simulink subsystem "Plant"  (R2024b)
settings: Solver=VariableStepAuto  StartTime=0.0  StopTime=10.0  RelTol=1e-3
undefined symbols (not defined in the file): body, wheels
settings Model: Creator=Marij  LastModifiedBy=marijn

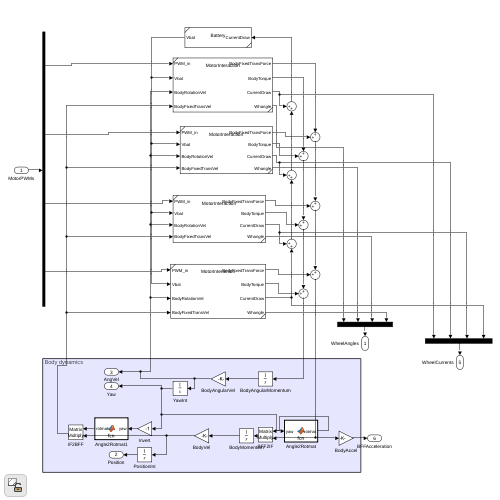
[thumbnail: Simulink's stored preview of the top-level diagram]
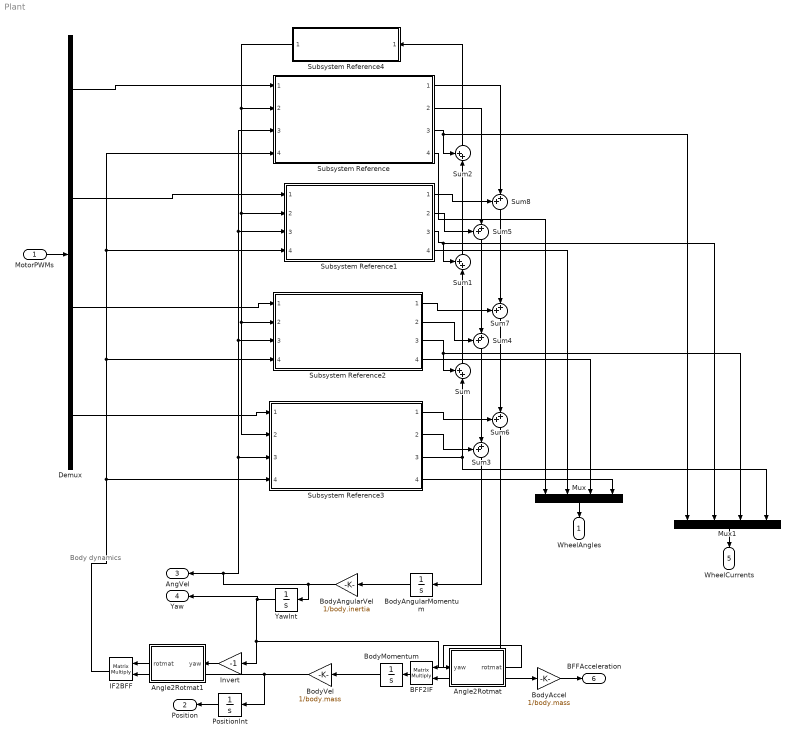
== system Plant ==
  note: Body dynamics
  MotorPWMs : Inport  PortDimensions=4
  Angle2Rotmat : MATLAB Function  TreatAsAtomicUnit=on
  Angle2Rotmat1 : MATLAB Function  TreatAsAtomicUnit=on
  BFF2IF : Product  Multiplication=Matrix(*)
  BodyAccel : Gain  Gain=1/body.mass
  BodyAngularMomentum : Integrator  ContinuousStateAttributes='AngularMomentum'
  BodyAngularVel : Gain  Gain=1/body.inertia
  BodyMomentum : Integrator  ContinuousStateAttributes={'XVelocity', 'YVelocity'}
  BodyVel : Gain  Gain=1/body.mass
  Demux : Demux
  IF2BFF : Product  Multiplication=Matrix(*)
  Invert : Gain  Gain=-1
  Mux : Mux
  Mux1 : Mux
  PositionInt : Integrator  ContinuousStateAttributes={'XPosition', 'YPosition'}
  Subsystem Reference : Subsystem  ReferencedSubsystem=MotorInteraction  whangle=wheels.angles(1)
  Subsystem Reference1 : Subsystem  ReferencedSubsystem=MotorInteraction  whangle=wheels.angles(2)
  Subsystem Reference2 : Subsystem  ReferencedSubsystem=MotorInteraction  whangle=wheels.angles(3)
  Subsystem Reference3 : Subsystem  ReferencedSubsystem=MotorInteraction  whangle=wheels.angles(4)
  Subsystem Reference4 : Subsystem  ReferencedSubsystem=Battery
  Sum{,1..8} (9 alike) : Sum  Inputs=++|
  YawInt : Integrator  ContinuousStateAttributes='Yaw'
  WheelAngles : Outport  Unit=rad  PortDimensions=4
  Position : Outport  Port=2  Unit=m  PortDimensions=2
  AngVel : Outport  Port=3  Unit=rad/s  PortDimensions=1
  Yaw : Outport  Port=4  Unit=rad  PortDimensions=1
  WheelCurrents : Outport  Port=5  Unit=A  PortDimensions=4
  BFFAcceleration : Outport  Port=6
  wires:
  YawInt/1 -> Yaw/1, Angle2Rotmat/1(yaw), Invert/1
  BodyAccel/1 -> BFFAcceleration/1
  Subsystem Reference4/1 -> Subsystem Reference/2, Subsystem Reference1/2, Subsystem Reference3/2, Subsystem Reference2/2
  Mux1/1 -> WheelCurrents/1
  Sum6/1 -> BodyAccel/1, BFF2IF/2
  Sum2/1 -> Subsystem Reference4/1
  Subsystem Reference3/4 -> Mux/4
  Subsystem Reference/4 -> Mux/1
  Sum3/1 -> BodyAngularMomentum/1
  Angle2Rotmat1/1(rotmat) -> IF2BFF/1
  BodyMomentum/1 -> BodyVel/1
  BodyVel/1 -> PositionInt/1, IF2BFF/2
  IF2BFF/1 -> Subsystem Reference2/4, Subsystem Reference1/4, Subsystem Reference/4, Subsystem Reference3/4
  Mux/1 -> WheelAngles/1
  BodyAngularMomentum/1 -> BodyAngularVel/1
  Subsystem Reference2/2 -> Sum4/1
  Subsystem Reference2/4 -> Mux/3
  Subsystem Reference/3 -> Mux1/1, Sum2/1
  PositionInt/1 -> Position/1
  MotorPWMs/1 -> Demux/1
  Sum/1 -> Sum1/2
  Subsystem Reference1/3 -> Mux1/2, Sum1/1
  Sum1/1 -> Sum2/2
  Demux/3 -> Subsystem Reference2/1
  Demux/4 -> Subsystem Reference3/1
  Subsystem Reference3/3 -> Mux1/4, Sum/2
  Demux/1 -> Subsystem Reference/1
  BodyAngularVel/1 -> YawInt/1, AngVel/1, Subsystem Reference3/3, Subsystem Reference2/3, Subsystem Reference1/3, Subsystem Reference/3
  Sum8/1 -> Sum7/2
  Sum4/1 -> Sum3/2
  Subsystem Reference1/4 -> Mux/2
  Angle2Rotmat/1(rotmat) -> BFF2IF/1
  BFF2IF/1 -> BodyMomentum/1
  Subsystem Reference2/3 -> Mux1/3, Sum/1
  Subsystem Reference1/1 -> Sum8/1
  Subsystem Reference3/2 -> Sum3/1
  Invert/1 -> Angle2Rotmat1/1(yaw)
  Subsystem Reference1/2 -> Sum5/1
  Subsystem Reference/1 -> Sum8/2
  Demux/2 -> Subsystem Reference1/1
  Subsystem Reference3/1 -> Sum6/1
  Subsystem Reference2/1 -> Sum7/1
  Sum7/1 -> Sum6/2
  Sum5/1 -> Sum4/2
  Subsystem Reference/2 -> Sum5/2

== matlab function Plant/Angle2Rotmat ==
  data: yaw input; rotmat output
function rotmat = fcn(yaw)
rotmat = [cos(yaw), -sin(yaw); sin(yaw), cos(yaw)];

== matlab function Plant/Angle2Rotmat1 ==
  data: yaw input; rotmat output
function rotmat = fcn(yaw)
rotmat = [cos(yaw), -sin(yaw); sin(yaw), cos(yaw)];
